simulink model "Analisis_espectro_R2018a"  (R2018a)
settings: Solver=VariableStepAuto  StartTime=0.0  StopTime=5  RelTol=1e-3
undefined symbols (not defined in the file): area_mem, c, k, m, perm, Q, r2, r_ambiente, rho, v_sonido, ventana_fft_analisis, zoh_freq_analisis
libraries: dspxfrm3 x2, dspvision x2, dspmtrx3 x2
settings Model: Creator=tobip  LastModifiedBy=tobip
settings DataIOCC: ReturnWorkspaceOutputs=on
settings DebuggingCC: UnconnectedInputMsg=none  UnconnectedOutputMsg=none  UnconnectedLineMsg=none
settings ModelReferenceCC: EnableRefExpFcnMdlSchedulingChecks=off
settings SFSimCC: SimUseLocalCustomCode=on
settings RTWCC: Description=Generic Real-Time Target  RTWUseLocalCustomCode=on

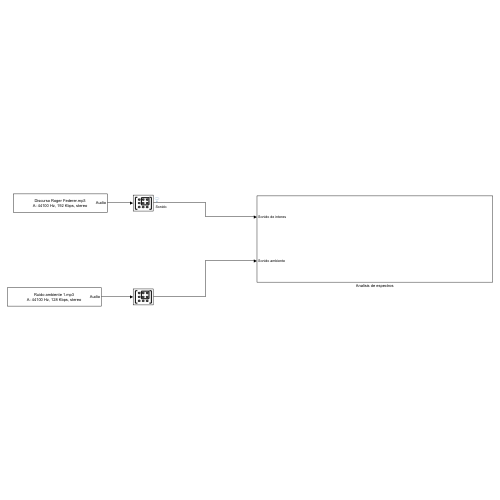
[thumbnail: Simulink's stored preview of the top-level diagram]
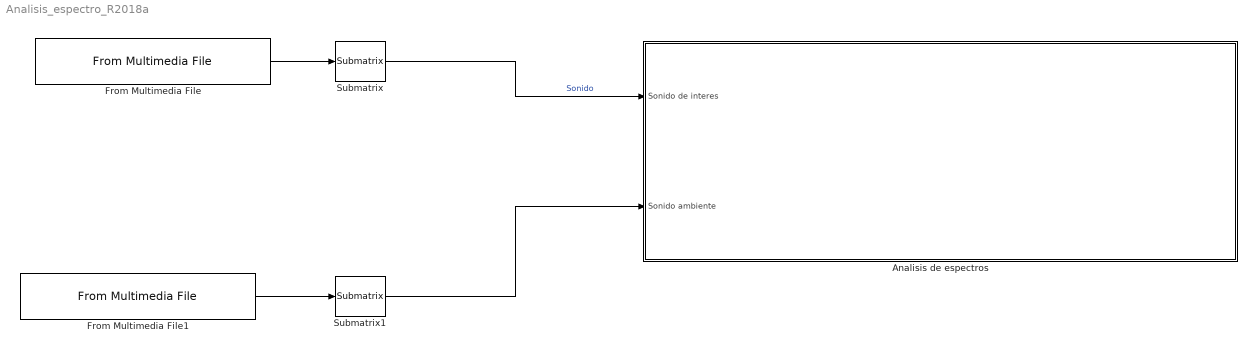
== system Analisis_espectro_R2018a ==
  Analisis de espectros : Subsystem
  From Multimedia File : dspvision/From Multimedia File  inputFilename=C:\Users\tobip\Documents\Control\Proyecto final\Discurso Roger Federer.mp3  loop=on  numPlays=1  outputStreams=Audio only  videoDataType=single  audioDataType=double  inheritSampleTime=on  userDefinedSampleTime=1/30  noAudioOutput=off  isIntensityVideo=off  fourcc=RGB  colorVideoFormat=Separate color signals  outputEOF=off  dataOrg=Column-major  audioFrameSize=1  computeAudioFrameSize=off  outSamplingMode=Sample based
  From Multimedia File1 : dspvision/From Multimedia File  inputFilename=C:\Users\tobip\Documents\Control\Proyecto final\Ruido ambiente 1.mp3  loop=on  numPlays=1  outputStreams=Audio only  videoDataType=single  audioDataType=double  inheritSampleTime=on  userDefinedSampleTime=1/30  noAudioOutput=off  isIntensityVideo=off  fourcc=RGB  colorVideoFormat=Separate color signals  outputEOF=off  dataOrg=Column-major  audioFrameSize=1  computeAudioFrameSize=off  outSamplingMode=Sample based
  Submatrix : dspmtrx3/Submatrix  RowSpan=All rows  RowStartMode=First  RowStartIndex=1  RowEndMode=Middle  RowEndIndex=1  ColSpan=One column  ColStartMode=First  ColStartIndex=1  ColEndMode=Last  ColEndIndex=1
  Submatrix1 : dspmtrx3/Submatrix  RowSpan=All rows  RowStartMode=First  RowStartIndex=1  RowEndMode=Last  RowEndIndex=1  ColSpan=One column  ColStartMode=First  ColStartIndex=1  ColEndMode=Last  ColEndIndex=1
  wires:
  From Multimedia File/1 -> Submatrix/1
  From Multimedia File1/1 -> Submatrix1/1
  Submatrix/1 -> Analisis de espectros/1(Sonido de interes)  "Sonido"
  Submatrix1/1 -> Analisis de espectros/2(Sonido ambiente)

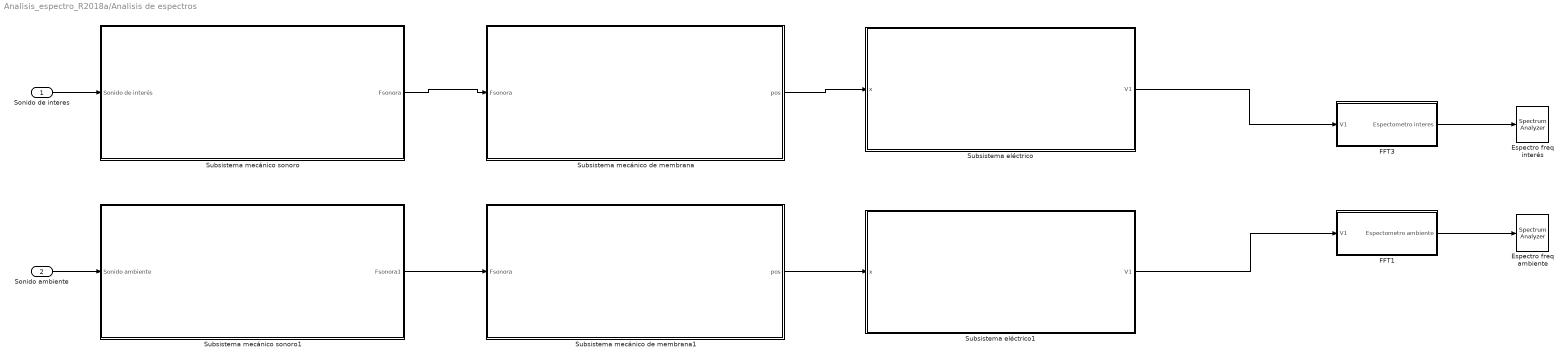
== system Analisis_espectro_R2018a/Analisis de espectros ==
  Sonido de interes : Inport
  Sonido ambiente : Inport  Port=2
  Espectro freq ambiente : SpectrumAnalyzer  DefaultConfigurationName=spbscopes.SpectrumAnalyzerBlockCfg
  Espectro freq interés : SpectrumAnalyzer  DefaultConfigurationName=spbscopes.SpectrumAnalyzerBlockCfg
  FFT1 : Subsystem
  FFT3 : Subsystem
  Subsistema eléctrico : Subsystem
  Subsistema eléctrico1 : Subsystem
  Subsistema mecánico de membrana : Subsystem
  Subsistema mecánico de membrana1 : Subsystem
  Subsistema mecánico sonoro : Subsystem
  Subsistema mecánico sonoro1 : Subsystem
  wires:
  Subsistema mecánico de membrana/1(pos) -> Subsistema eléctrico/1(x)
  Sonido de interes/1 -> Subsistema mecánico sonoro/1(Sonido de interés)
  Subsistema eléctrico/1(V1) -> FFT3/1(V1)
  Subsistema mecánico sonoro/1(Fsonora) -> Subsistema mecánico de membrana/1(Fsonora)
  Sonido ambiente/1 -> Subsistema mecánico sonoro1/1(Sonido ambiente)
  Subsistema eléctrico1/1(V1) -> FFT1/1(V1)
  Subsistema mecánico de membrana1/1(pos) -> Subsistema eléctrico1/1(x)
  Subsistema mecánico sonoro1/1(Fsonora1) -> Subsistema mecánico de membrana1/1(Fsonora)
  FFT3/1(Espectometro interes) -> Espectro freq interés/1
  FFT1/1(Espectometro ambiente) -> Espectro freq ambiente/1

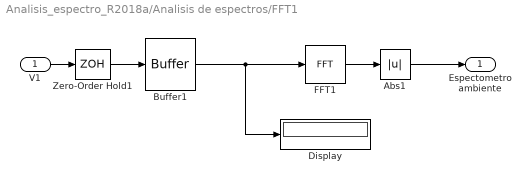
== system Analisis_espectro_R2018a/Analisis de espectros/FFT1 ==
  V1 : Inport
  Abs1 : Abs
  Buffer1 : Buffer  N=ventana_fft_analisis  V=ventana_fft_analisis-1  OutputFrames=off
  Display : Display
  FFT1 : dspxfrm3/FFT  FFTImplementation=Auto  CompMethod=Table lookup  TableOpt=NEW  TableOptActive=Speed  BitRevOrder=off  Normalize=off  InheritFFTLength=on  FFTLength=64  WrapInput=on  roundingMode=Floor  overflowMode=off  firstCoeffDataTypeStr=Inherit: Same word length as input  firstCoeffLastDataTypeStr=Inherit: Same word length as input  outputMin=[]  outputMax=[]
  Zero-Order Hold1 : ZeroOrderHold  SampleTime=zoh_freq_analisis
  Espectometro ambiente : Outport
  wires:
  V1/1 -> Zero-Order Hold1/1
  Zero-Order Hold1/1 -> Buffer1/1
  FFT1/1 -> Abs1/1
  Abs1/1 -> Espectometro ambiente/1
  Buffer1/1 -> Display/1, FFT1/1

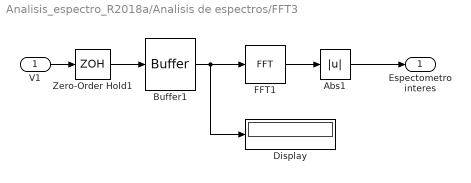
== system Analisis_espectro_R2018a/Analisis de espectros/FFT3 ==
  V1 : Inport
  Abs1 : Abs
  Buffer1 : Buffer  N=ventana_fft_analisis  V=ventana_fft_analisis-1  OutputFrames=off
  Display : Display
  FFT1 : dspxfrm3/FFT  FFTImplementation=Auto  CompMethod=Table lookup  TableOpt=NEW  TableOptActive=Speed  BitRevOrder=off  Normalize=off  InheritFFTLength=on  FFTLength=64  WrapInput=on  roundingMode=Floor  overflowMode=off  firstCoeffDataTypeStr=Inherit: Same word length as input  firstCoeffLastDataTypeStr=Inherit: Same word length as input  outputMin=[]  outputMax=[]
  Zero-Order Hold1 : ZeroOrderHold  SampleTime=zoh_freq_analisis
  Espectometro interes : Outport
  wires:
  V1/1 -> Zero-Order Hold1/1
  Zero-Order Hold1/1 -> Buffer1/1
  FFT1/1 -> Abs1/1
  Abs1/1 -> Espectometro interes/1
  Buffer1/1 -> Display/1, FFT1/1

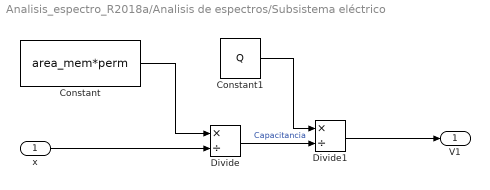
== system Analisis_espectro_R2018a/Analisis de espectros/Subsistema eléctrico ==
  x : Inport
  Constant : Constant  Value=area_mem*perm
  Constant1 : Constant  Value=Q
  Divide : Product  Inputs=*/
  Divide1 : Product  Inputs=*/
  V1 : Outport
  wires:
  x/1 -> Divide/2
  Constant/1 -> Divide/1
  Divide/1 -> Divide1/2  "Capacitancia"
  Divide1/1 -> V1/1
  Constant1/1 -> Divide1/1

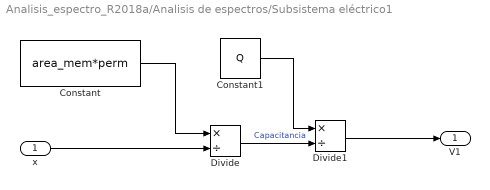
== system Analisis_espectro_R2018a/Analisis de espectros/Subsistema eléctrico1 ==
  x : Inport
  Constant : Constant  Value=area_mem*perm
  Constant1 : Constant  Value=Q
  Divide : Product  Inputs=*/
  Divide1 : Product  Inputs=*/
  V1 : Outport
  wires:
  x/1 -> Divide/2
  Constant/1 -> Divide/1
  Divide/1 -> Divide1/2  "Capacitancia"
  Divide1/1 -> V1/1
  Constant1/1 -> Divide1/1

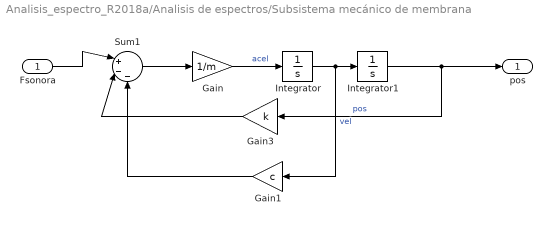
== system Analisis_espectro_R2018a/Analisis de espectros/Subsistema mecánico de membrana ==
  Fsonora : Inport
  Gain : Gain  Gain=1/m
  Gain1 : Gain  Gain=c
  Gain3 : Gain  Gain=k
  Integrator : Integrator
  Integrator1 : Integrator
  Sum1 : Sum  Inputs=|+--
  pos : Outport
  wires:
  Integrator1/1 -> Gain3/1, pos/1  "pos"
  Integrator/1 -> Gain1/1, Integrator1/1  "vel"
  Fsonora/1 -> Sum1/1
  Gain3/1 -> Sum1/2
  Sum1/1 -> Gain/1
  Gain/1 -> Integrator/1  "acel"
  Gain1/1 -> Sum1/3

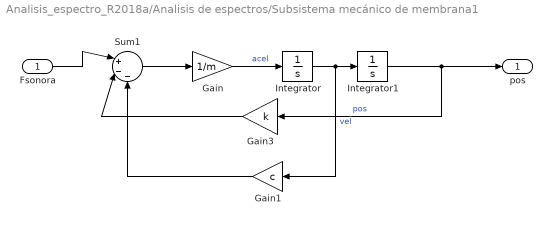
== system Analisis_espectro_R2018a/Analisis de espectros/Subsistema mecánico de membrana1 ==
  Fsonora : Inport
  Gain : Gain  Gain=1/m
  Gain1 : Gain  Gain=c
  Gain3 : Gain  Gain=k
  Integrator : Integrator
  Integrator1 : Integrator
  Sum1 : Sum  Inputs=|+--
  pos : Outport
  wires:
  Integrator1/1 -> Gain3/1, pos/1  "pos"
  Integrator/1 -> Gain1/1, Integrator1/1  "vel"
  Fsonora/1 -> Sum1/1
  Gain3/1 -> Sum1/2
  Sum1/1 -> Gain/1
  Gain/1 -> Integrator/1  "acel"
  Gain1/1 -> Sum1/3

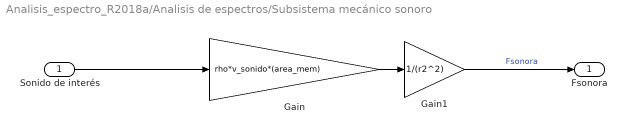
== system Analisis_espectro_R2018a/Analisis de espectros/Subsistema mecánico sonoro ==
  Sonido de interés : Inport
  Gain : Gain  Gain=rho*v_sonido*(area_mem)
  Gain1 : Gain  Gain=1/(r2^2)
  Fsonora : Outport
  wires:
  Gain/1 -> Gain1/1
  Sonido de interés/1 -> Gain/1
  Gain1/1 -> Fsonora/1  "Fsonora"

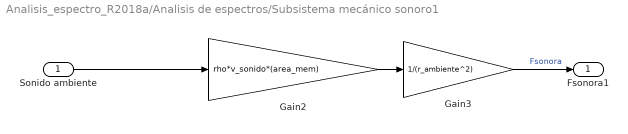
== system Analisis_espectro_R2018a/Analisis de espectros/Subsistema mecánico sonoro1 ==
  Sonido ambiente : Inport
  Gain2 : Gain  Gain=rho*v_sonido*(area_mem)
  Gain3 : Gain  Gain=1/(r_ambiente^2)
  Fsonora1 : Outport
  wires:
  Gain2/1 -> Gain3/1
  Gain3/1 -> Fsonora1/1  "Fsonora"
  Sonido ambiente/1 -> Gain2/1
